simulink model "process_model_1"  (R2023b)
settings: Solver=FixedStepDiscrete  StartTime=0.0  StopTime=10.0  RelTol=1e-3
values from neighbouring files (symbols this model uses):
  a_1 = 0.9897    [ca2_params.m]    (also in iterate_gains.m)
  b_1 = 0.05263    [ca2_params.m]    (also in iterate_gains.m)
  d_1 = 15    [ca2_params.m]    (also in iterate_gains.m)
  samp_t = 1    [ca2_params.m]    (also in iterate_gains.m)
settings Model: Creator=john  LastModifiedBy=john

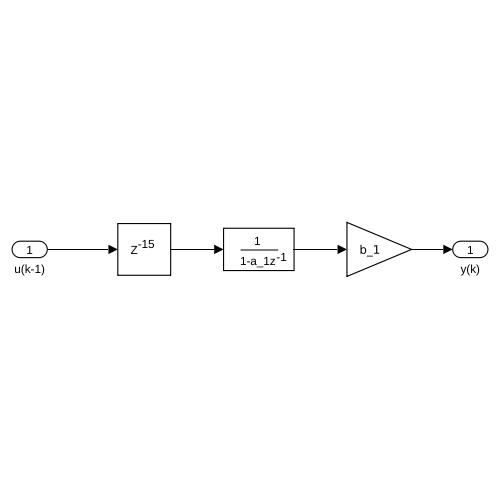
[thumbnail: Simulink's stored preview of the top-level diagram]
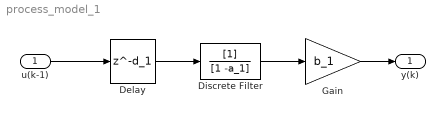
== system process_model_1 ==
  u(k-1) : Inport
  Delay : Delay  DelayLength=d_1  SampleTime=samp_t
  Discrete Filter : DiscreteFilter  Denominator=[1 -a_1]
  Gain : Gain  Gain=b_1
  y(k) : Outport
  wires:
  Delay/1 -> Discrete Filter/1
  u(k-1)/1 -> Delay/1
  Discrete Filter/1 -> Gain/1
  Gain/1 -> y(k)/1
